simulink model "pb1"  (R2020b)
settings: Solver=VariableStepAuto  StartTime=0.0  StopTime=10.0  RelTol=1e-3
undefined symbols (not defined in the file): b, k1, k2, m1, m2
settings Model: Creator=Hinal  LastModifiedBy=Hinal

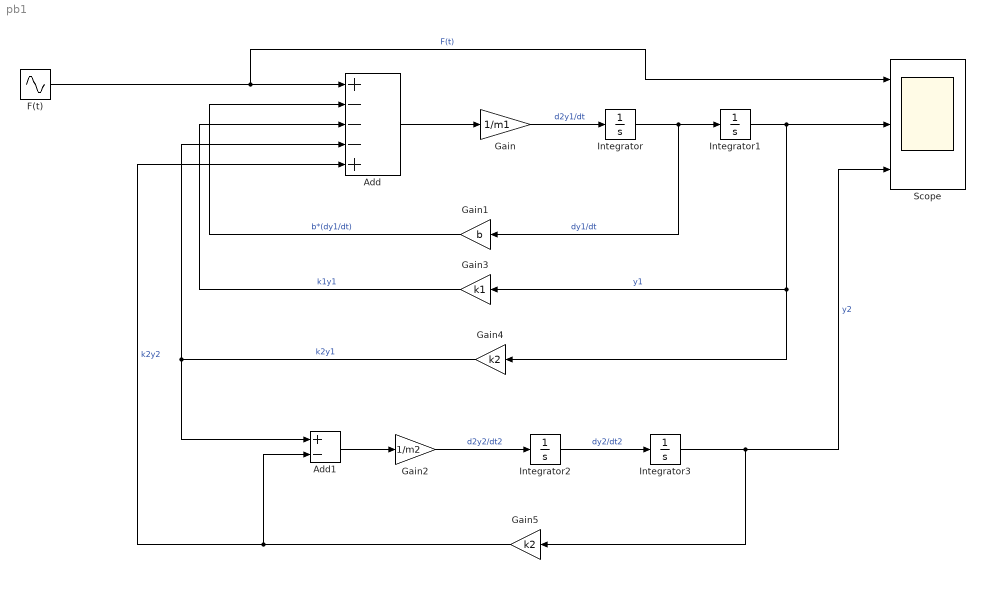
== system pb1 ==
  Add : Sum  Inputs=+---+
  Add1 : Sum  Inputs=+-
  F(t) : Sin  Amplitude=2  Frequency=10  SampleTime=0
  Gain : Gain  Gain=1/m1
  Gain1 : Gain  Gain=b
  Gain2 : Gain  Gain=1/m2
  Gain3 : Gain  Gain=k1
  Gain4 : Gain  Gain=k2
  Gain5 : Gain  Gain=k2
  Integrator{,1..3} (4 alike) : Integrator
  Scope : Scope  NumInputPorts=3
  wires:
  Add1/1 -> Gain2/1
  Gain2/1 -> Integrator2/1  "d2y2/dt2"
  Integrator3/1 -> Scope/3, Gain5/1  "y2"
  F(t)/1 -> Scope/1, Add/1  "F(t)"
  Gain5/1 -> Add1/2, Add/5  "k2y2"
  Gain4/1 -> Add1/1, Add/4  "k2y1"
  Integrator2/1 -> Integrator3/1  "dy2/dt2"
  Gain1/1 -> Add/2  "b*(dy1/dt)"
  Gain3/1 -> Add/3  "k1y1"
  Integrator/1 -> Gain1/1, Integrator1/1  "dy1/dt"
  Gain/1 -> Integrator/1  "d2y1/dt"
  Add/1 -> Gain/1
  Integrator1/1 -> Gain4/1, Gain3/1, Scope/2  "y1"
